simulink model "hvac_1zone_v3"  (R2021a)
settings: Solver=FixedStepAuto  StartTime=0.0  StopTime=Inf  FixedStep=2  RelTol=1e-3  EnableMultiTasking=on
values from neighbouring files (symbols this model uses):
  Ts2 = 600    [main_1zone.m]
  V = load('values1z.mat')    [main_1zone.m]
undefined symbols (not defined in the file or in its folder): den, num, rl
libraries: dspmathops x1, rllib x1
settings Model: Creator=User  LastModifiedBy=Richi
settings SolverCC: AlgebraicLoopSolver=TrustRegion
settings DataIOCC: LimitDataPoints=on  SaveFormat=Array  SignalLoggingSaveFormat=ModelDataLogs
settings OptimizationCC: LifeSpan=inf
settings DebuggingCC: SolverPrmCheckMsg=warning  MultiTaskDSMMsg=warning  MultiTaskCondExecSysMsg=none  MultiTaskRateTransMsg=warning  AllowSymbolicDim=off  SFUnexpectedBacktrackingDiag=warning  SFNoUnconditionalDefaultTransitionDiag=warning  SFExecutionAtInitializationDiag=none  SFMachineParentedDataDiag=warning  ArithmeticOperatorsInVariantConditions=warning
settings HardwareCC: ProdBitPerPointer=32  ProdBitPerSizeT=32  ProdBitPerPtrDiffT=32  ProdLargestAtomicFloat=None  ProdIntDivRoundTo=Undefined  ProdEndianess=Unspecified  ProdWordSize=32  ProdHWDeviceType=32-bit Generic
settings ModelReferenceCC: PropagateSignalLabelsOutOfModel=off
settings SFSimCC: SimUseLocalCustomCode=off  CustomCodeUndefinedFunction=UseInterfaceOnly
settings RTWCC: RTWUseLocalCustomCode=off
settings CodeAppCC: StateflowObjectComments=on
settings GRTTargetCC: TargetLangStandard=C89/C90 (ANSI)
settings ConfigComp: CovMetricSettings=dw  CovSaveCumulativeToWorkspaceVar=on  CovSaveSingleToWorkspaceVar=on  CovExternalEMLEnable=off

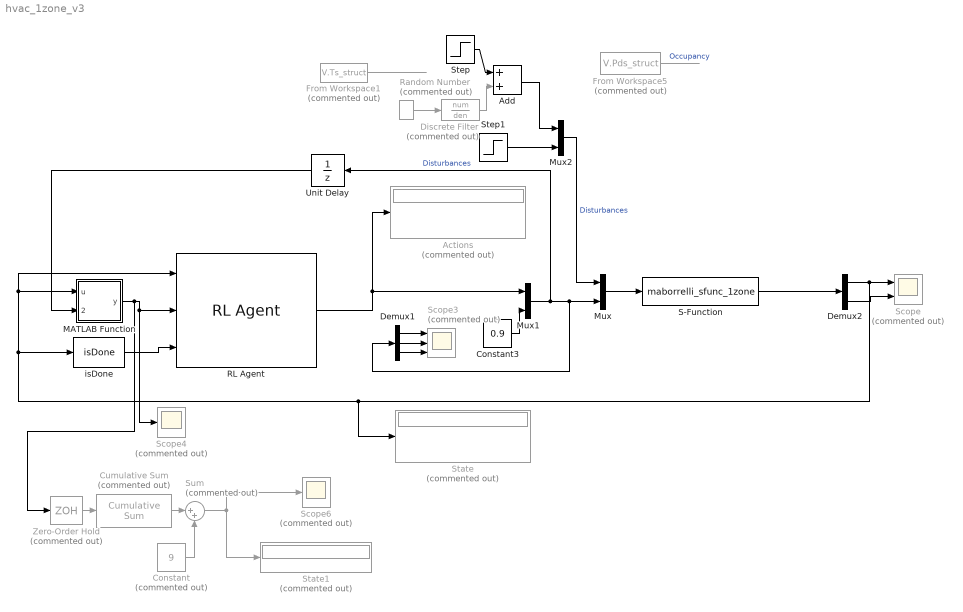
== system hvac_1zone_v3 ==
  Actions : Display  Commented=on
  Add : Sum
  Constant : Constant  Commented=on  Value=9
  Constant3 : Constant  Value=0.9
  Cumulative Sum : dspmathops/Cumulative Sum  Commented=on  dim=Channels (running sum)  InputProcessing=Columns as channels (frame based)  reset_popup=None  roundingMode=Floor  overflowMode=off  outputDataTypeStr=Inherit: Same as accumulator  outputMin=[]  outputMax=[]  outputLastDataTypeStr=Inherit: Same as accumulator
  Demux1 : Demux  Outputs=3
  Demux2 : Demux  Outputs=2
  Discrete Filter : DiscreteFilter  Commented=on  Numerator=num  Denominator=den  SampleTime=5400
  From Workspace1 : FromWorkspace  Commented=on  VariableName=V.Ts_struct  OutDataTypeStr=double  SampleTime=-1
  From Workspace5 : FromWorkspace  Commented=on  VariableName=V.Pds_struct  OutDataTypeStr=double  SampleTime=-1
  MATLAB Function : MATLAB Function  TreatAsAtomicUnit=on
  Mux : Mux  Inputs=2
  Mux1 : Mux  Inputs=2
  Mux2 : Mux  Inputs=2
  RL Agent : rllib/RL Agent  Agent=rl.util.PolicyInstance.get('hvac_1zone_v3/RL Agent')  ExternalActionAsInput=off  ProvideCumRwd=off  TreatAsDirectFeedthrough=on
  Random Number : RandomNumber  Commented=on  Variance=0.5  SampleTime=1800
  S-Function : S-Function  FunctionName=maborrelli_sfunc_1zone  Parameters=[34;34],V.params1,60  SFunctionDeploymentMode=off  EnableBusSupport=off
  Scope : Scope  Commented=on  NumInputPorts=2
  Scope3 : Scope  Commented=on  NumInputPorts=3
  Scope4 : Scope  Commented=on
  Scope6 : Scope  Commented=on
  State : Display  Commented=on
  State1 : Display  Commented=on
  Step : Step  Before=40  After=40  SampleTime=0
  Step1 : Step  Before=200  After=200  SampleTime=0
  Sum : Sum  Commented=on  Inputs=|++
  Unit Delay : UnitDelay  SampleTime=Ts2  HasFrameUpgradeWarning=on
  Zero-Order Hold : ZeroOrderHold  Commented=on  SampleTime=Ts2
  isDone : M-S-Function  FunctionName=isDone
  wires:
  Mux2/1 -> Mux/1  "Disturbances"
  From Workspace5/1 -> ?  "Occupancy"
  Mux/1 -> S-Function/1
  Discrete Filter/1 -> Add/2
  Add/1 -> Mux2/1
  Random Number/1 -> Discrete Filter/1
  RL Agent/1 -> Actions/1, Mux1/1
  isDone/1 -> RL Agent/3
  MATLAB Function/1(y) -> Zero-Order Hold/1, Scope4/1, RL Agent/2
  Demux1/2 -> Scope3/2
  Demux1/1 -> Scope3/1
  Demux1/3 -> Scope3/3
  Demux2/2 -> Scope/2
  S-Function/1 -> Demux2/1
  Mux1/1 -> Unit Delay/1, Demux1/1, Mux/2  "Disturbances"
  Constant3/1 -> Mux1/2
  Unit Delay/1 -> MATLAB Function/2(actions)
  Cumulative Sum/1 -> Sum/1
  Zero-Order Hold/1 -> Cumulative Sum/1
  Sum/1 -> State1/1, Scope6/1
  Constant/1 -> Sum/2
  From Workspace1/1 -> ?
  Demux2/1 -> isDone/1, RL Agent/1, MATLAB Function/1(u), State/1, Scope/1
  Step/1 -> Add/1
  Step1/1 -> Mux2/2

== matlab function hvac_1zone_v3/MATLAB Function ==
  data: u input; y output; actions input
function y = reward(u, actions)
 low = 22;
 high = 25;
 ms = actions(1);
 Dt = actions(2);
 %Añadir energía:
 e = ((-1012/4)*ms*Dt+ 65*(ms)^2)*2.7778e-04;
 reward = -0.8 * e; 
 %disp(length(block.InputPort(1).Data))
 for i=1:1
     %disp(i)
     aux = u(i);
     %disp(aux)
     if (aux < low || aux > high) && (abs(aux - low) >= 1 && abs(aux-high) >= 1)
        %disp(abs(aux - low))
        reward = reward - min( abs(aux - low), abs(aux - high));
        %reward = reward + 0;
        %disp('if13')
     end
     %disp('if1')
     %if (aux >= low && aux <= high)
     %   reward = reward + 0.5;
     %end

 end
y = reward;
